simulink model "week3problem1"  (R2020b)
settings: Solver=VariableStepAuto  StartTime=0.0  StopTime=10.0  RelTol=1e-3
settings Model: Creator=Puru Gawande  LastModifiedBy=Puru Gawande

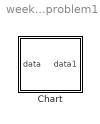
== system week3problem1 ==
  Chart : Stateflow chart  TreatAsAtomicUnit=on

== stateflow chart week3problem1/Chart ==
  state Got_0
  state Got_Nickel
  state Got_Dime
  (default) -> Got_0
  Got_0 -> Got_Nickel [order 1] : [data1==1]{data=0}
  Got_Nickel -> Got_0 [order 1] : [data1==2]{data=1}
  Got_Dime -> Got_0 [order 2] : [data1==1]{data=1}
  Got_0 -> Got_Dime [order 2] : [data1==2]{data=0}
  Got_Nickel -> Got_Dime [order 2] : [data1==1]{data=0}
  Got_Dime -> Got_Nickel [order 1] : [data1==2]{data=1}
  data: data input; data1 output
